simulink model "Powertrain_Simulation"  (R2021b)
settings: Solver=VariableStepAuto  StartTime=0.0  StopTime=time_in_s(end)  RelTol=1e-3
values from neighbouring files (symbols this model uses):
  A = 3751 * 0.00064516    (= 2.41999516)    [Master_Script.m]
  acc_power = 2    [Master_Script.m]
  Cd = 0.38    [Master_Script.m]
  den = 1.21    [Master_Script.m]
  eff_batt = 0.9    [Master_Script.m]
  eff_generator = 0.85    [Master_Script.m]
  eff_motor = 0.85    [Master_Script.m]
  eff_transmission = 0.95    [Master_Script.m]
  EM_torque_Nm = EM_torque_Nm * 3    [Master_Script.m]
  fr = 0.015    [Master_Script.m]
  g = 9.81    [Master_Script.m]
  gas_den = 0.74    [Master_Script.m]
  gear_ratio = 8    [Master_Script.m]
  m = 4428*0.453592    (= 2008.505376)    [Master_Script.m]
  mass_flow_rate = 0.01    [Master_Script.m]
  MaxTrac = u * m * (a*g+h*MaxAcc) / wheelbase / 1000    (= 15.5282117967)    [Master_Script.m]
  R = 364/1000    (= 0.364)    [Master_Script.m]
  spd_time_in_s = time_in_s    [Master_Script.m]
  spd_velocity = velocity_in_mph    [Master_Script.m]
  useDriveCycle = 1    [Master_Script.m]
undefined symbols (not defined in the file or in its folder): alpha, batt, EM_RPM, eng
libraries: simulink x3, slpidlib x1
settings Model: Creator=Rajdeep Pawar  LastModifiedBy=Shubham
settings DebuggingCC: AlgebraicLoopMsg=none

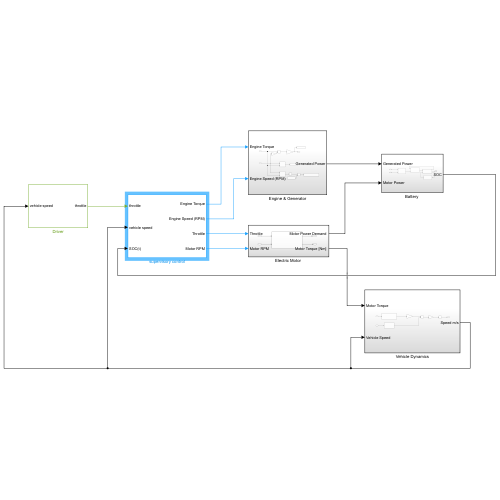
[thumbnail: Simulink's stored preview of the top-level diagram]
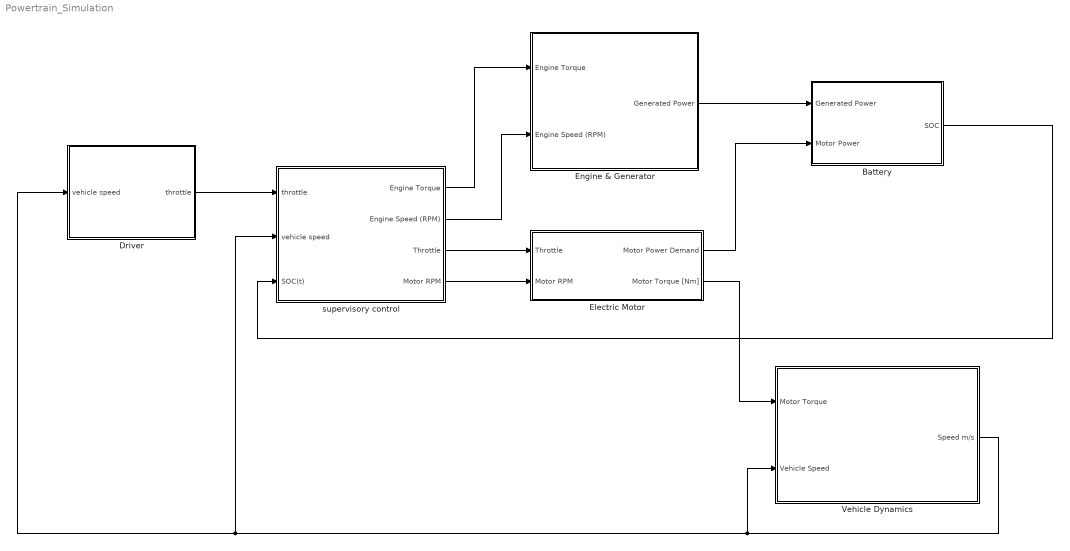
== system Powertrain_Simulation ==
  "Battery " : Subsystem
  Driver : Subsystem
  "Electric Motor " : Subsystem
  Engine & Generator : Subsystem
  Vehicle Dynamics : Subsystem
  supervisory control : Subsystem
  wires:
  Driver/1(throttle) -> supervisory control/1(throttle)
  supervisory control/1(Engine Torque) -> Engine & Generator/1(Engine Torque)
  supervisory control/2(Engine Speed (RPM)) -> Engine & Generator/2(Engine Speed (RPM))
  "Battery "/1(SOC) -> supervisory control/3(SOC(t))
  supervisory control/3(Throttle) -> "Electric Motor "/1(Throttle)
  supervisory control/4(Motor RPM) -> "Electric Motor "/2(Motor RPM)
  Engine & Generator/1(Generated Power) -> "Battery "/1(Generated Power)
  "Electric Motor "/1("Motor Power Demand ") -> "Battery "/2(Motor Power)
  "Electric Motor "/2("Motor Torque [Nm] ") -> Vehicle Dynamics/1(Motor Torque)
  Vehicle Dynamics/1(Speed m/s) -> Vehicle Dynamics/2(Vehicle Speed), supervisory control/2(vehicle speed), Driver/1(vehicle speed)

== system Powertrain_Simulation/Battery  ==
  Generated Power : Inport
  Motor Power : Inport  Port=2
  "Battery " : Subsystem
  Battery Current : Subsystem
  Battery Management System : Subsystem
  Net Power : Subsystem
  SOC : Outport
  wires:
  Battery Management System/1(T_cell) -> "Battery "/2(T_cell_in_C)  "T_cell"
  "Battery "/1(Terminal Voltage) -> Battery Current/1(Vt)
  Battery Current/1(Current Demand) -> "Battery "/1(Current)
  "Battery "/3(Q_dot_gen) -> Battery Management System/1(Q_dot_gen)
  "Battery "/2(SOC) -> SOC/1
  Generated Power/1 -> Net Power/1(Generated Power)  "Engine Power"
  Motor Power/1 -> Net Power/2(Motor Power)  "Motor Power"
  Net Power/1(Net Power) -> Battery Current/2(Net Power)

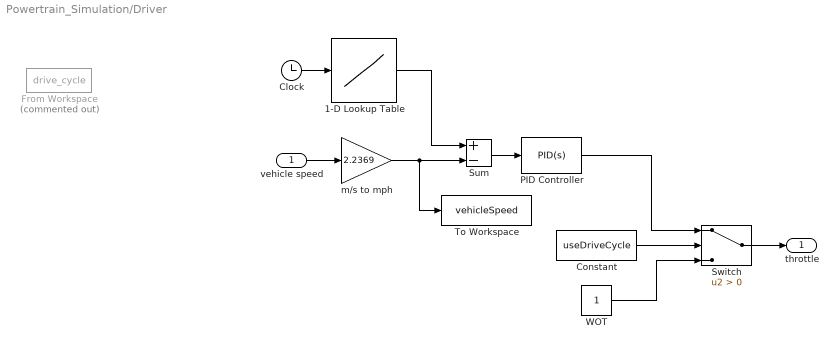
== system Powertrain_Simulation/Driver ==
  vehicle speed : Inport
  1-D Lookup Table : Lookup_n-D  NumberOfTableDimensions=1  BreakpointsForDimension1=spd_time_in_s  Table=spd_velocity  InternalRulePriority=Speed  RndMeth=Simplest  InputSameDT=on
  Clock : Clock
  Constant : Constant  Value=useDriveCycle
  From Workspace : FromWorkspace  Commented=on  VariableName=drive_cycle
  PID Controller : slpidlib/PID Controller  Controller=PID  Form=Parallel  TimeDomain=Continuous-time  UseExternalTs=off  SampleTime=-1  IntegratorMethod=Forward Euler  FilterMethod=Forward Euler  ControllerParametersSource=internal  P=1  I=0  D=0  UseFilter=on  N=100  TunerSelectOption=Transfer Function Based (PID Tuner App)  InitialConditionSource=internal  InitialConditionForIntegrator=0  InitialConditionForFilter=0  DifferentiatorICPrevScaledInput=0  ExternalReset=none  TrackingMode=off  Kt=1  LimitOutput=on  SatLimitsSource=internal  UpperSaturationLimit=1  LowerSaturationLimit=-1  LinearizeAsGain=on  AntiWindupMode=none  Kb=1  POutMin=[]  POutMax=[]  IOutMin=[]  IOutMax=[]  DOutMin=[]  DOutMax=[]  NOutMin=[]  NOutMax=[]  SumOutMin=[]  SumOutMax=[]  SaturationOutMin=[]  SaturationOutMax=[]  PParamMin=[]  PParamMax=[]  IParamMin=[]  IParamMax=[]  DParamMin=[]  DParamMax=[]  NParamMin=[]  NParamMax=[]  KbParamMin=[]  KbParamMax=[]  KtParamMin=[]  KtParamMax=[]  KbOutMin=[]  KbOutMax=[]  KtOutMin=[]  KtOutMax=[]  IntegratorOutMin=[]  IntegratorOutMax=[]  FilterOutMin=[]  FilterOutMax=[]  SumI1OutMin=[]  SumI1OutMax=[]  SumI2OutMin=[]  SumI2OutMax=[]  SumI3OutMin=[]  SumI3OutMax=[]  SumI4OutMin=[]  SumI4OutMax=[]  SumDOutMin=[]  SumDOutMax=[]  DifferentiatorOutMin=[]  DifferentiatorOutMax=[]  FilterDiffOutCoefMin=[]  FilterDiffOutCoefMax=[]  ReciprocalOutMin=[]  ReciprocalOutMax=[]  SumDenOutMin=[]  SumDenOutMax=[]  SumNumOutMin=[]  SumNumOutMax=[]  DivideOutMin=[]  DivideOutMax=[]  UdiffTsProdOutMin=[]  UdiffTsProdOutMax=[]  NTsProdOutMin=[]  NTsProdOutMax=[]  UintegralTsProdOutMin=[]  UintegralTsProdOutMax=[]  UngainTsProdOutMin=[]  UngainTsProdOutMax=[]  IntegratorContinuousStateAttributes=''  IntegratorStateMustResolveToSignalObject=off  IntegratorRTWStateStorageClass=Auto  FilterContinuousStateAttributes=''  FilterStateMustResolveToSignalObject=off  FilterRTWStateStorageClass=Auto  ParallelPVariant=InternalParameters  IdealPVariant=Disabled  IVariant=InternalParameters  DVariant=InternalParameters  IntegratorVariant=Continuous  SatVariant=Enabled  AWVariant=Passthrough  PCopyVariant=Disabled  TRVariant=Disabled  FdbkBlocksVariant=Forward  IdealPFdbkVariant=Disabled  SatFdbkVariant=Disabled  DerivativeFilterVariant=ContFilter  NVariant=InternalParameters  NCopyVariant=Disabled  FilterICVariant=InternalICsFilter  IntegratorICVariant=InternalICs  ExternalResetVariant=Disabled  TRSumVariant=Passthrough  SumFdbkVariant=Disabled  SumVariant=Sum_PID  TsampFilterVariant=InternalTs  TsampNgainVariant=Passthrough  TsampIntegralVariant=Passthrough  ExternalSaturationOutDataTypeStr=Inherit: Same as second input
  Sum : Sum  Inputs=+-
  Switch : Switch  Criteria=u2 > Threshold
  To Workspace : ToWorkspace  VariableName=vehicleSpeed  SaveFormat=Timeseries  SampleTime=-1
  WOT : Constant
  m/s to mph : Gain  Gain=2.2369
  throttle : Outport
  wires:
  Sum/1 -> PID Controller/1
  vehicle speed/1 -> m/s to mph/1
  Switch/1 -> throttle/1
  PID Controller/1 -> Switch/1
  WOT/1 -> Switch/3
  Constant/1 -> Switch/2
  Clock/1 -> 1-D Lookup Table/1
  m/s to mph/1 -> To Workspace/1, Sum/2
  1-D Lookup Table/1 -> Sum/1

== system Powertrain_Simulation/Electric Motor  ==
  Throttle : Inport
  Motor RPM : Inport  Port=2
  Electric motor model : Subsystem
  "Motor Power Demand " : Outport
  "Motor Torque [Nm] " : Outport  Port=2
  wires:
  Electric motor model/1("Motor Torque [Nm] ") -> "Motor Torque [Nm] "/1
  Throttle/1 -> Electric motor model/1("Throttle [-1 to 1] ")
  Motor RPM/1 -> Electric motor model/2(Motor speed [RPM])
  Electric motor model/2(Motor Power Demand [W]) -> "Motor Power Demand "/1

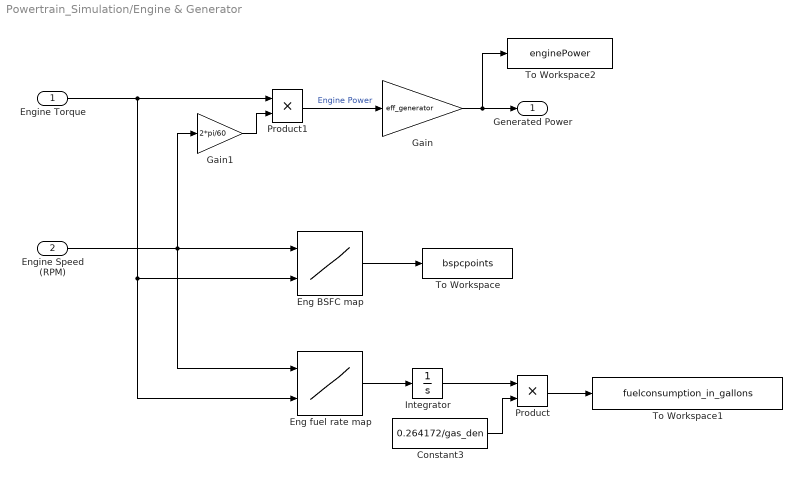
== system Powertrain_Simulation/Engine & Generator ==
  Engine Torque : Inport
  Engine Speed (RPM) : Inport  Port=2
  Constant3 : Constant  Value=0.264172/gas_den
  Eng BSFC map : Lookup_n-D  BreakpointsForDimension1=eng.BSFC.RPM  BreakpointsForDimension2=eng.BSFC.T  Table=eng.BSFC.BSFC  InternalRulePriority=Speed  RndMeth=Simplest  InputSameDT=on
      settings: InputPortMap=u0,u1
  Eng fuel rate map : Lookup_n-D  BreakpointsForDimension1=eng.BSFC.RPM  BreakpointsForDimension2=eng.BSFC.T  Table=eng.BSFC.fuel_rate  InternalRulePriority=Speed  RndMeth=Simplest  InputSameDT=on
      settings: InputPortMap=u0,u1
  Gain : Gain  Gain=eff_generator
  Gain1 : Gain  Gain=2*pi/60
  Integrator : Integrator
  Product : Product
  Product1 : Product
  To Workspace : ToWorkspace  VariableName=bspcpoints  SaveFormat=Timeseries  SampleTime=-1
  To Workspace1 : ToWorkspace  VariableName=fuelconsumption_in_gallons  SampleTime=-1
  To Workspace2 : ToWorkspace  VariableName=enginePower  SaveFormat=Timeseries  SampleTime=-1
  Generated Power : Outport
  wires:
  Engine Speed (RPM)/1 -> Gain1/1, Eng BSFC map/1, Eng fuel rate map/1
  Eng BSFC map/1 -> To Workspace/1
  Engine Torque/1 -> Eng fuel rate map/2, Eng BSFC map/2, Product1/1
  Integrator/1 -> Product/1
  Product/1 -> To Workspace1/1
  Constant3/1 -> Product/2
  Eng fuel rate map/1 -> Integrator/1
  Product1/1 -> Gain/1  "Engine Power"
  Gain/1 -> To Workspace2/1, Generated Power/1
  Gain1/1 -> Product1/2

== system Powertrain_Simulation/Vehicle Dynamics ==
  Motor Torque : Inport
  Vehicle Speed : Inport  Port=2
  Gain : Gain  Gain=1/m
  Gain1 : Gain  Gain=gear_ratio/R
  Integrator : Integrator  InitialCondition=0.1
  Road Load : Subsystem
  Subtract : Sum  Inputs=+-
  Transmission efficiency : Subsystem
  Speed m/s : Outport
  wires:
  Gain/1 -> Integrator/1  "acceleration"
  Integrator/1 -> Speed m/s/1  "speed m/s"
  Vehicle Speed/1 -> Road Load/1(velocity)
  Motor Torque/1 -> Transmission efficiency/1(torque at trans. in)
  Gain1/1 -> Subtract/1  "Traction Force"
  Road Load/1(Road Load (N)) -> Subtract/2
  Subtract/1 -> Gain/1
  Transmission efficiency/1(torque at trans. out) -> Gain1/1  "Torque at Gearbox output"

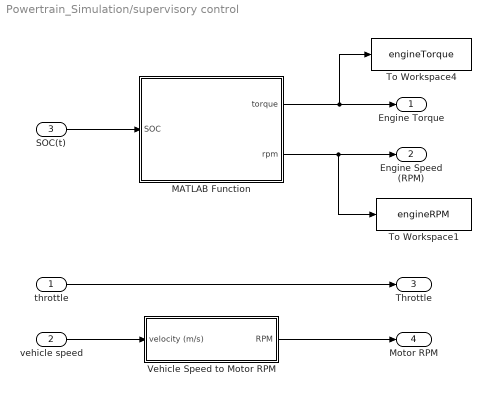
== system Powertrain_Simulation/supervisory control ==
  throttle : Inport
  vehicle speed : Inport  Port=2
  SOC(t) : Inport  Port=3
  MATLAB Function : MATLAB Function  TreatAsAtomicUnit=on
  To Workspace1 : ToWorkspace  VariableName=engineRPM  SampleTime=-1
  To Workspace4 : ToWorkspace  VariableName=engineTorque  SampleTime=-1
  Vehicle Speed to Motor RPM : Subsystem
  Engine Torque : Outport
  Engine Speed (RPM) : Outport  Port=2
  Throttle : Outport  Port=3
  Motor RPM : Outport  Port=4
  wires:
  throttle/1 -> Throttle/1
  Vehicle Speed to Motor RPM/1(RPM) -> Motor RPM/1
  SOC(t)/1 -> MATLAB Function/1(SOC)
  vehicle speed/1 -> Vehicle Speed to Motor RPM/1(velocity (m/s))
  MATLAB Function/2(rpm) -> Engine Speed (RPM)/1, To Workspace1/1
  MATLAB Function/1(torque) -> To Workspace4/1, Engine Torque/1

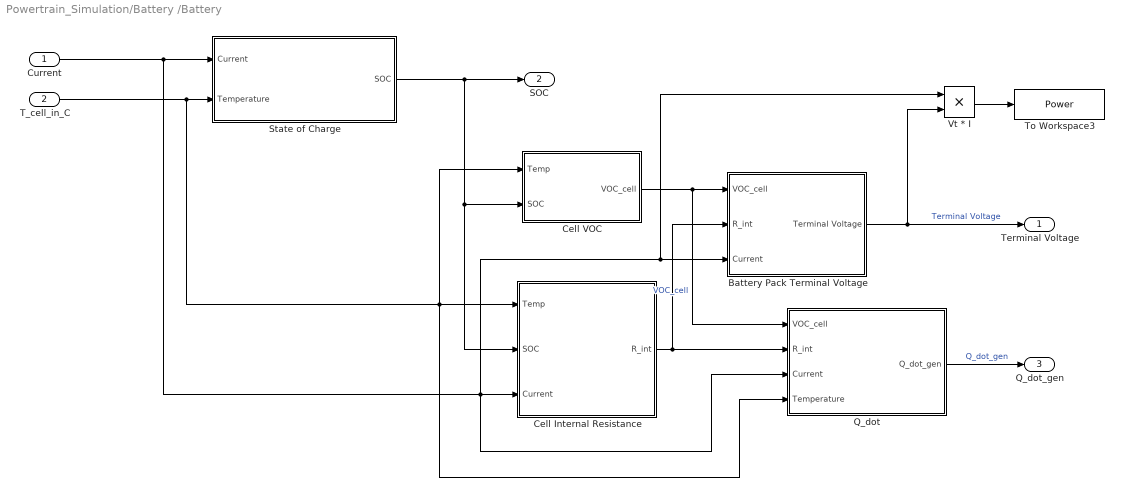
== system Powertrain_Simulation/Battery /Battery  ==
  Current : Inport
  T_cell_in_C : Inport  Port=2
  Battery Pack Terminal Voltage : Subsystem
  Cell Internal Resistance : Subsystem
  Cell VOC : Subsystem
  Q_dot : Subsystem
  State of Charge : Subsystem
  To Workspace3 : ToWorkspace  VariableName=Power  SaveFormat=Timeseries  SampleTime=-1
  Vt * I : Product
  Terminal Voltage : Outport
  SOC : Outport  Port=2
  Q_dot_gen : Outport  Port=3
  wires:
  Current/1 -> State of Charge/1(Current), Vt * I/1, Battery Pack Terminal Voltage/3(Current), Q_dot/3(Current), Cell Internal Resistance/3(Current)
  Vt * I/1 -> To Workspace3/1
  State of Charge/1(SOC) -> SOC/1, Cell Internal Resistance/2(SOC), Cell VOC/2(SOC)
  Battery Pack Terminal Voltage/1(Terminal Voltage) -> Vt * I/2, Terminal Voltage/1  "Terminal Voltage"
  Cell VOC/1(VOC_cell) -> Q_dot/1(VOC_cell), Battery Pack Terminal Voltage/1(VOC_cell)  "VOC_cell"
  Q_dot/1(Q_dot_gen) -> Q_dot_gen/1  "Q_dot_gen"
  T_cell_in_C/1 -> Cell VOC/1(Temp), Q_dot/4(Temperature), Cell Internal Resistance/1(Temp), State of Charge/2(Temperature)
  Cell Internal Resistance/1(R_int) -> Battery Pack Terminal Voltage/2(R_int), Q_dot/2(R_int)

== system Powertrain_Simulation/Battery /Battery Current ==
  Vt : Inport
  Net Power : Inport  Port=2
  Constant : Constant  Value=batt.curr_chg_max
  Constant1 : Constant  Value=batt.curr_dis_max
  Divide1 : Product  Inputs=*/
  Saturation Dynamic1 : simulink/Discontinuities/Saturation Dynamic  OutMin=[]  OutMax=[]  OutDataTypeStr=Inherit: Same as second input  OutDataType=fixdt(1, 16)  OutScaling=2^-10  DoSatur=off
  To Workspace : ToWorkspace  VariableName=current  SaveFormat=Timeseries  SampleTime=-1
  Current Demand : Outport
  wires:
  Divide1/1 -> Saturation Dynamic1/2  "Current"
  Constant1/1 -> Saturation Dynamic1/1
  Saturation Dynamic1/1 -> To Workspace/1, Current Demand/1  "Current Demand"
  Constant/1 -> Saturation Dynamic1/3
  Net Power/1 -> Divide1/1
  Vt/1 -> Divide1/2

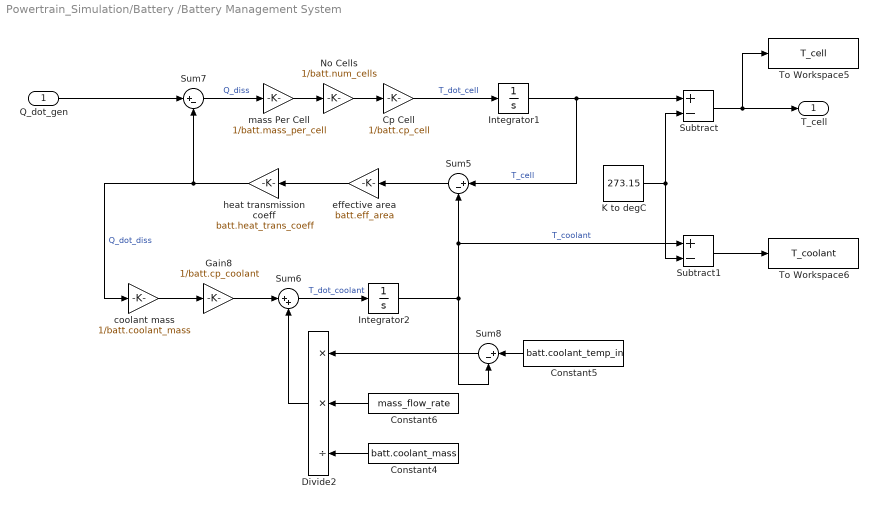
== system Powertrain_Simulation/Battery /Battery Management System ==
  Q_dot_gen : Inport
  Constant4 : Constant  Value=batt.coolant_mass
  Constant5 : Constant  Value=batt.coolant_temp_in
  Constant6 : Constant  Value=mass_flow_rate
  Cp Cell : Gain  Gain=1/batt.cp_cell
  Divide2 : Product  Inputs=**/
  Gain8 : Gain  Gain=1/batt.cp_coolant
  Integrator1 : Integrator  InitialCondition=batt.amb_temp
  Integrator2 : Integrator  InitialCondition=batt.coolant_temp_in
  K to degC : Constant  Value=273.15
  No Cells : Gain  Gain=1/batt.num_cells
  Subtract : Sum  Inputs=+-
  Subtract1 : Sum  Inputs=+-
  Sum5 : Sum  Inputs=|+-
  Sum6 : Sum  Inputs=|++
  Sum7 : Sum  Inputs=|+-
  Sum8 : Sum  Inputs=|+-
  To Workspace5 : ToWorkspace  VariableName=T_cell  SaveFormat=Timeseries  SampleTime=-1
  To Workspace6 : ToWorkspace  VariableName=T_coolant  SaveFormat=Timeseries  SampleTime=-1
  coolant mass : Gain  Gain=1/batt.coolant_mass
  effective area : Gain  Gain=batt.eff_area
  heat transmission coeff : Gain  Gain=batt.heat_trans_coeff
  mass Per Cell : Gain  Gain=1/batt.mass_per_cell
  T_cell : Outport
  wires:
  Sum5/1 -> effective area/1
  Integrator2/1 -> Sum5/2, Subtract1/1, Sum8/2  "T_coolant"
  Integrator1/1 -> Sum5/1, Subtract/1  "T_cell"
  Constant5/1 -> Sum8/1
  coolant mass/1 -> Gain8/1
  heat transmission coeff/1 -> Sum7/2, coolant mass/1  "Q_dot_diss"
  Cp Cell/1 -> Integrator1/1  "T_dot_cell"
  effective area/1 -> heat transmission coeff/1
  Sum7/1 -> mass Per Cell/1  "Q_diss"
  Divide2/1 -> Sum6/2
  Constant4/1 -> Divide2/3
  Gain8/1 -> Sum6/1
  Sum8/1 -> Divide2/1
  Sum6/1 -> Integrator2/1  "T_dot_coolant"
  Constant6/1 -> Divide2/2
  Q_dot_gen/1 -> Sum7/1
  mass Per Cell/1 -> No Cells/1
  No Cells/1 -> Cp Cell/1
  K to degC/1 -> Subtract/2, Subtract1/2
  Subtract/1 -> To Workspace5/1, T_cell/1
  Subtract1/1 -> To Workspace6/1

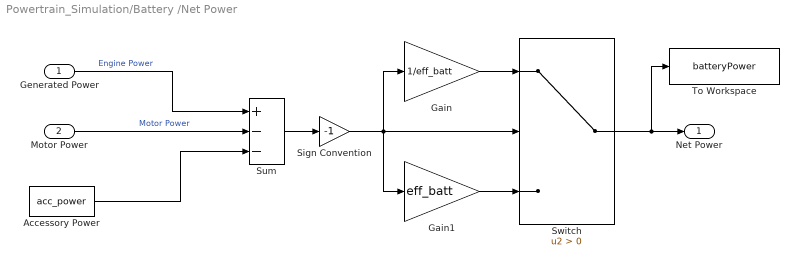
== system Powertrain_Simulation/Battery /Net Power ==
  Generated Power : Inport
  Motor Power : Inport  Port=2
  Accessory Power : Constant  Value=acc_power
  Gain : Gain  Gain=1/eff_batt
  Gain1 : Gain  Gain=eff_batt
  Sign Convention : Gain  Gain=-1
  Sum : Sum  Inputs=+--
  Switch : Switch  Criteria=u2 > Threshold
  To Workspace : ToWorkspace  VariableName=batteryPower  SaveFormat=Timeseries  SampleTime=-1
  Net Power : Outport
  wires:
  Generated Power/1 -> Sum/1  "Engine Power"
  Sum/1 -> Sign Convention/1
  Motor Power/1 -> Sum/2  "Motor Power"
  Sign Convention/1 -> Gain1/1, Gain/1, Switch/2
  Gain/1 -> Switch/1
  Gain1/1 -> Switch/3
  Accessory Power/1 -> Sum/3
  Switch/1 -> To Workspace/1, Net Power/1

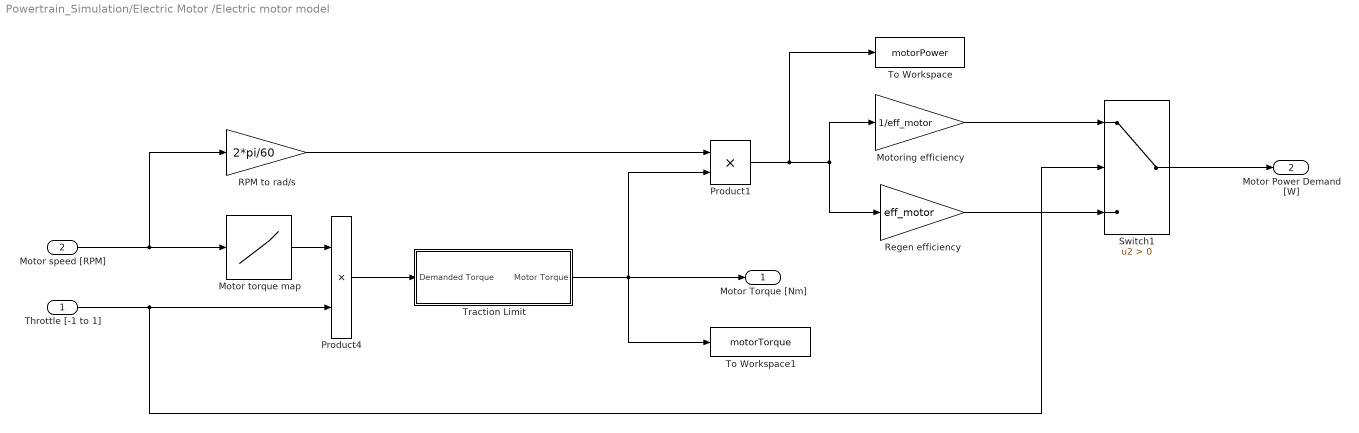
== system Powertrain_Simulation/Electric Motor /Electric motor model ==
  "Throttle [-1 to 1] " : Inport
  Motor speed [RPM] : Inport  Port=2
  Motor torque map : Lookup_n-D  NumberOfTableDimensions=1  BreakpointsForDimension1=EM_RPM  BreakpointsForDimension2=alpha  Table=EM_torque_Nm  InternalRulePriority=Speed  RndMeth=Simplest  InputSameDT=on
  Motoring efficiency : Gain  Gain=1/eff_motor
  Product1 : Product
  Product4 : Product  RndMeth=Zero
  RPM to rad/s : Gain  Gain=2*pi/60
  Regen efficiency : Gain  Gain=eff_motor
  Switch1 : Switch  Criteria=u2 > Threshold
  To Workspace : ToWorkspace  VariableName=motorPower  SaveFormat=Timeseries  SampleTime=-1
  To Workspace1 : ToWorkspace  VariableName=motorTorque  SaveFormat=Timeseries  SampleTime=-1
  Traction Limit : Subsystem
  "Motor Torque [Nm] " : Outport
  Motor Power Demand [W] : Outport  Port=2
  wires:
  Motor torque map/1 -> Product4/1
  RPM to rad/s/1 -> Product1/1
  Motor speed [RPM]/1 -> RPM to rad/s/1, Motor torque map/1
  Motoring efficiency/1 -> Switch1/1
  Regen efficiency/1 -> Switch1/3
  "Throttle [-1 to 1] "/1 -> Switch1/2, Product4/2
  Switch1/1 -> Motor Power Demand [W]/1
  Product1/1 -> To Workspace/1, Motoring efficiency/1, Regen efficiency/1
  Product4/1 -> Traction Limit/1(Demanded Torque)
  Traction Limit/1(Motor Torque) -> To Workspace1/1, "Motor Torque [Nm] "/1, Product1/2

== system Powertrain_Simulation/Vehicle Dynamics/Road Load ==
  velocity : Inport
  Add : Sum
  Air Resistance : Subsystem
  Rolling Resistance : Subsystem
  Road Load (N) : Outport
  wires:
  velocity/1 -> Rolling Resistance/1(velocity), Air Resistance/1(velocity)
  Air Resistance/1(Air Drag) -> Add/1
  Rolling Resistance/1(Roll Resistance) -> Add/2
  Add/1 -> Road Load (N)/1

== system Powertrain_Simulation/Vehicle Dynamics/Transmission efficiency ==
  torque at trans. in : Inport
  Transmission Efficiency : Gain  Gain=eff_transmission
  torque at trans. out : Outport
  wires:
  torque at trans. in/1 -> Transmission Efficiency/1
  Transmission Efficiency/1 -> torque at trans. out/1

== system Powertrain_Simulation/supervisory control/Vehicle Speed to Motor RPM ==
  velocity (m/s) : Inport
  Gain2 : Gain  Gain=1/R
  Gain3 : Gain  Gain=gear_ratio
  rad/s to RPM : Gain  Gain=60/(2*pi)
  RPM : Outport
  wires:
  Gain3/1 -> rad/s to RPM/1
  Gain2/1 -> Gain3/1
  velocity (m/s)/1 -> Gain2/1
  rad/s to RPM/1 -> RPM/1

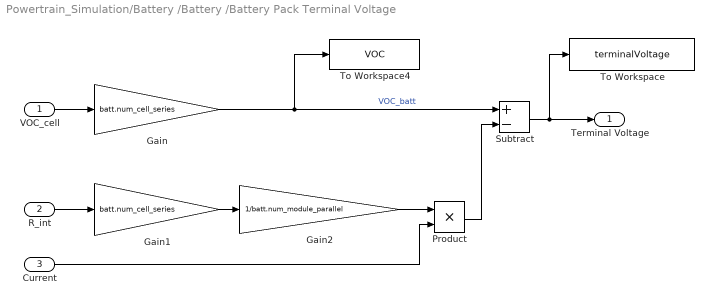
== system Powertrain_Simulation/Battery /Battery /Battery Pack Terminal Voltage ==
  VOC_cell : Inport
  R_int : Inport  Port=2
  Current : Inport  Port=3
  Gain : Gain  Gain=batt.num_cell_series
  Gain1 : Gain  Gain=batt.num_cell_series
  Gain2 : Gain  Gain=1/batt.num_module_parallel
  Product : Product
  Subtract : Sum  Inputs=+-  OutMin=batt.volt_min/batt.num_cell_series  OutMax=batt.volt_max/batt.num_cell_series
  To Workspace : ToWorkspace  VariableName=terminalVoltage  SaveFormat=Timeseries  SampleTime=-1
  To Workspace4 : ToWorkspace  VariableName=VOC  SaveFormat=Timeseries  SampleTime=-1
  Terminal Voltage : Outport
  wires:
  R_int/1 -> Gain1/1
  Current/1 -> Product/2
  Product/1 -> Subtract/2
  Subtract/1 -> Terminal Voltage/1, To Workspace/1
  VOC_cell/1 -> Gain/1
  Gain/1 -> Subtract/1, To Workspace4/1  "VOC_batt"
  Gain1/1 -> Gain2/1
  Gain2/1 -> Product/1

== system Powertrain_Simulation/Battery /Battery /Cell Internal Resistance ==
  Temp : Inport
  SOC : Inport  Port=2
  Current : Inport  Port=3
  Charge : Lookup_n-D  BreakpointsForDimension1=batt.r_int_chg.temp  BreakpointsForDimension2=batt.r_int_chg.soc  Table=batt.r_int_chg.r_int  InternalRulePriority=Speed  RndMeth=Simplest  InputSameDT=on
      settings: InputPortMap=u0,u1
  Discharge : Lookup_n-D  BreakpointsForDimension1=batt.r_int_dis.temp  BreakpointsForDimension2=batt.r_int_dis.soc  Table=batt.r_int_dis.r_int  InternalRulePriority=Speed  RndMeth=Simplest  InputSameDT=on
      settings: InputPortMap=u0,u1
  Switch : Switch
  R_int : Outport
  wires:
  Current/1 -> Switch/2
  Temp/1 -> Discharge/1, Charge/1
  SOC/1 -> Discharge/2, Charge/2
  Charge/1 -> Switch/3
  Discharge/1 -> Switch/1
  Switch/1 -> R_int/1

== system Powertrain_Simulation/Battery /Battery /Cell VOC ==
  Temp : Inport
  SOC : Inport  Port=2
  Constant2 : Constant  Value=batt.volt_max
  Constant3 : Constant  Value=batt.volt_min
  Saturation Dynamic2 : simulink/Discontinuities/Saturation Dynamic  OutMin=[]  OutMax=[]  OutDataTypeStr=Inherit: Same as second input  OutDataType=fixdt(1, 16)  OutScaling=2^-10  DoSatur=off
  voc : Lookup_n-D  BreakpointsForDimension1=batt.voc.temp  BreakpointsForDimension2=batt.voc.soc  Table=batt.voc.voc  InternalRulePriority=Speed  RndMeth=Simplest  InputSameDT=on
      settings: InputPortMap=u0,u1
  VOC_cell : Outport
  wires:
  voc/1 -> Saturation Dynamic2/2  "VOC"
  Constant2/1 -> Saturation Dynamic2/1
  Constant3/1 -> Saturation Dynamic2/3
  Saturation Dynamic2/1 -> VOC_cell/1  "Voc Single Cell"
  Temp/1 -> voc/1
  SOC/1 -> voc/2

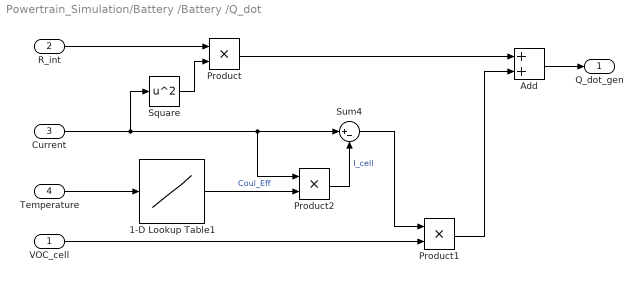
== system Powertrain_Simulation/Battery /Battery /Q_dot ==
  VOC_cell : Inport
  R_int : Inport  Port=2
  Current : Inport  Port=3
  Temperature : Inport  Port=4
  1-D Lookup Table1 : Lookup_n-D  NumberOfTableDimensions=1  BreakpointsForDimension1=batt.col_eff.temperature  Table=batt.col_eff.col_eff  InternalRulePriority=Speed  RndMeth=Simplest  InputSameDT=on
  Add : Sum
  Product : Product
  Product1 : Product
  Product2 : Product
  Square : Math  Operator=square  SaturateOnIntegerOverflow=on
  Sum4 : Sum  Inputs=|+-
  Q_dot_gen : Outport
  wires:
  1-D Lookup Table1/1 -> Product2/2  "Coul_Eff"
  Product2/1 -> Sum4/2  "I_cell"
  Sum4/1 -> Product1/1
  Current/1 -> Square/1, Sum4/1, Product2/1
  VOC_cell/1 -> Product1/2
  Square/1 -> Product/2
  R_int/1 -> Product/1
  Product/1 -> Add/1
  Product1/1 -> Add/2
  Add/1 -> Q_dot_gen/1
  Temperature/1 -> 1-D Lookup Table1/1

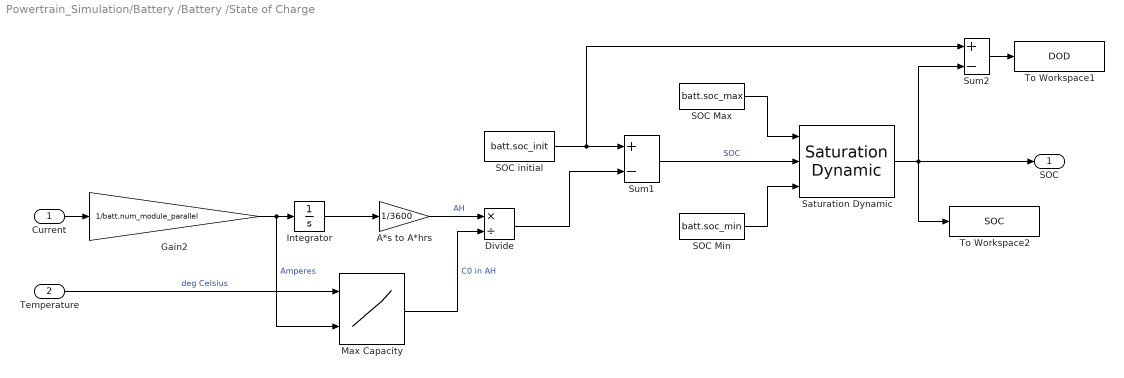
== system Powertrain_Simulation/Battery /Battery /State of Charge ==
  Current : Inport
  Temperature : Inport  Port=2
  A*s to A*hrs : Gain  Gain=1/3600
  Divide : Product  Inputs=*/
  Gain2 : Gain  Gain=1/batt.num_module_parallel
  Integrator : Integrator
  Max Capacity : Lookup_n-D  BreakpointsForDimension1=batt.cap_max.temp  BreakpointsForDimension2=batt.cap_max.curr  Table=batt.cap_max.cap_max  InternalRulePriority=Speed  RndMeth=Simplest  InputSameDT=on
      settings: InputPortMap=u0,u1
  SOC Max : Constant  Value=batt.soc_max
  SOC Min : Constant  Value=batt.soc_min
  "SOC initial " : Constant  Value=batt.soc_init
  Saturation Dynamic : simulink/Discontinuities/Saturation Dynamic  OutMin=[]  OutMax=[]  OutDataTypeStr=Inherit: Same as second input  OutDataType=fixdt(1, 16)  OutScaling=2^-10  DoSatur=off
  Sum1 : Sum  Inputs=+-
  Sum2 : Sum  Inputs=+-
  To Workspace1 : ToWorkspace  VariableName=DOD  SaveFormat=Timeseries  SampleTime=-1
  To Workspace2 : ToWorkspace  VariableName=SOC  SaveFormat=Timeseries  SampleTime=-1
  SOC : Outport
  wires:
  Max Capacity/1 -> Divide/2  "C0 in AH"
  A*s to A*hrs/1 -> Divide/1  "AH"
  Divide/1 -> Sum1/2
  Integrator/1 -> A*s to A*hrs/1
  SOC Max/1 -> Saturation Dynamic/1
  SOC Min/1 -> Saturation Dynamic/3
  Temperature/1 -> Max Capacity/1  "deg Celsius"
  Sum2/1 -> To Workspace1/1
  "SOC initial "/1 -> Sum2/1, Sum1/1
  Sum1/1 -> Saturation Dynamic/2  "SOC"
  Saturation Dynamic/1 -> Sum2/2, To Workspace2/1, SOC/1
  Current/1 -> Gain2/1
  Gain2/1 -> Max Capacity/2, Integrator/1  "Amperes"

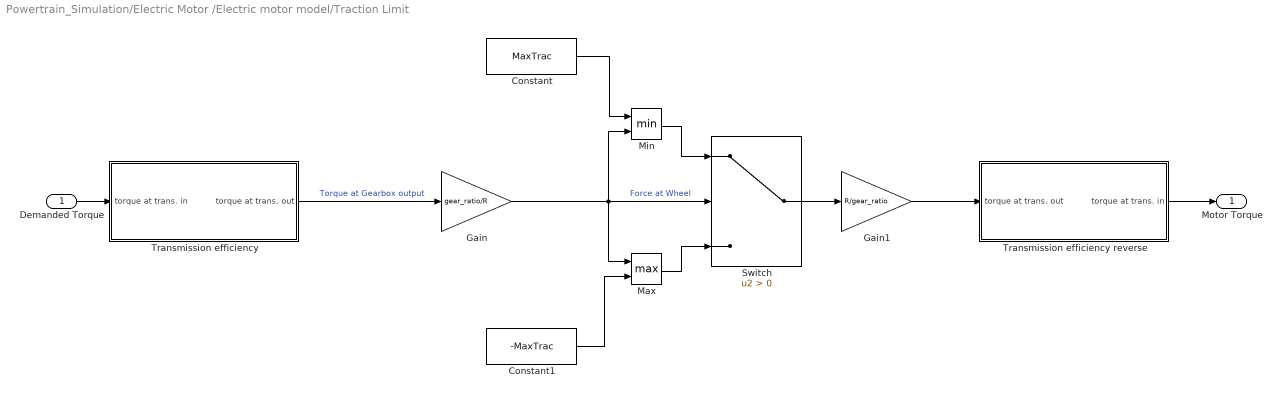
== system Powertrain_Simulation/Electric Motor /Electric motor model/Traction Limit ==
  Demanded Torque : Inport
  Constant : Constant  Value=MaxTrac
  Constant1 : Constant  Value=-MaxTrac
  Gain : Gain  Gain=gear_ratio/R
  Gain1 : Gain  Gain=R/gear_ratio
  Max : MinMax  Function=max  Inputs=2
  Min : MinMax  Inputs=2
  Switch : Switch  Criteria=u2 > Threshold
  Transmission efficiency : Subsystem
  Transmission efficiency reverse : Subsystem
  Motor Torque : Outport
  wires:
  Gain/1 -> Max/1, Min/2, Switch/2  "Force at Wheel"
  Constant/1 -> Min/1
  Min/1 -> Switch/1
  Gain1/1 -> Transmission efficiency reverse/1(torque at trans. out)
  Constant1/1 -> Max/2
  Max/1 -> Switch/3
  Switch/1 -> Gain1/1
  Demanded Torque/1 -> Transmission efficiency/1(torque at trans. in)
  Transmission efficiency/1(torque at trans. out) -> Gain/1  "Torque at Gearbox output"
  Transmission efficiency reverse/1(torque at trans. in) -> Motor Torque/1

== system Powertrain_Simulation/Vehicle Dynamics/Road Load/Air Resistance ==
  velocity : Inport
  Gain : Gain  Gain=den*Cd*A/2
  Square : Math  Operator=square  SaturateOnIntegerOverflow=on
  To Workspace2 : ToWorkspace  VariableName=aero_drag  SaveFormat=Timeseries  SampleTime=-1
  Air Drag : Outport
  wires:
  velocity/1 -> Square/1
  Square/1 -> Gain/1
  Gain/1 -> To Workspace2/1, Air Drag/1

== system Powertrain_Simulation/Vehicle Dynamics/Road Load/Rolling Resistance ==
  velocity : Inport
  Constant : Constant  Value=m
  Constant1 : Constant  Value=0
  Gain : Gain  Gain=g
  Gain1 : Gain  Gain=fr
  Switch : Switch  Criteria=u2 > Threshold
  Roll Resistance : Outport
  wires:
  Constant/1 -> Gain/1
  Gain/1 -> Gain1/1
  velocity/1 -> Switch/2
  Gain1/1 -> Switch/1
  Constant1/1 -> Switch/3
  Switch/1 -> Roll Resistance/1

== system Powertrain_Simulation/Electric Motor /Electric motor model/Traction Limit/Transmission efficiency ==
  torque at trans. in : Inport
  Transmission Efficiency : Gain  Gain=eff_transmission
  torque at trans. out : Outport
  wires:
  torque at trans. in/1 -> Transmission Efficiency/1
  Transmission Efficiency/1 -> torque at trans. out/1

== system Powertrain_Simulation/Electric Motor /Electric motor model/Traction Limit/Transmission efficiency reverse ==
  torque at trans. out : Inport
  Transmission Efficiency : Gain  Gain=1/eff_transmission
  torque at trans. in : Outport
  wires:
  torque at trans. out/1 -> Transmission Efficiency/1
  Transmission Efficiency/1 -> torque at trans. in/1

== matlab function Powertrain_Simulation/supervisory control/MATLAB Function ==
  data: SOC input; torque output; rpm output
function [torque, rpm] = engineOperationPoint(SOC)
%     if SOC > 0.95
%         torque = 10;    %// Accessory torque
%         rpm = 750;      %// Idling
%     elseif SOC > 0.7
%         torque = 35.74 * 4;
%         rpm = 2500;
%     elseif SOC > 0.4
%         torque = 35.74 * 4;
%         rpm = 2500;
%     else
%         torque = 127.16;
%         rpm = 6100;
%     end
    if(SOC > 0)
        torque = 140;
        rpm = 3700;
    end
    torque = 140;
    rpm = 3700;
end
